simulink subsystem "HIL"  (R2024a)
settings: Solver=VariableStepAuto  StartTime=0.0  StopTime=10.0  RelTol=1e-3
values from neighbouring files (symbols this model uses):
  Hil = 100.0    [ModelDD.sldd]
  Sim : value not decoded    [ModelDD.sldd]
undefined symbols (not defined in the file or in its folder): D1, Delta, DiscIntNeverNeededParam
libraries: simulink x60, spsSeriesRLCBranchLib x18, spsControlledVoltageSourceLib x15, spsThreePhaseVIMeasurementLib x9, spsGroundLib x8, hdlsllib x6, spsMosfetLib x6, spsabctodq0Lib x5, spsDCVoltageSourceLib x3, spsPower3phInstantaneousLib x3, spsVoltageMeasurementLib x3, spspowerguiLib x3
(part 1 of 3)
settings Model: Creator=The Professionals  LastModifiedBy=The Professionals

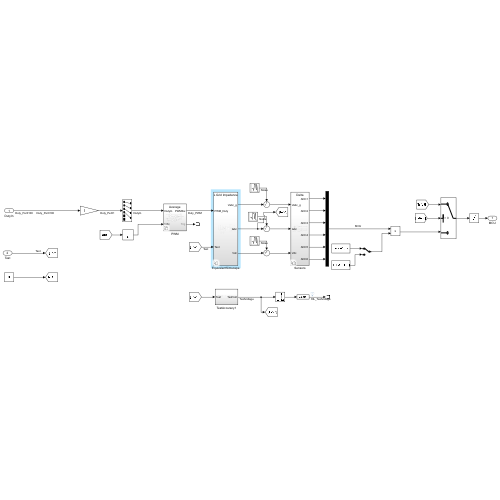
[thumbnail: Simulink's stored preview of the top-level diagram]
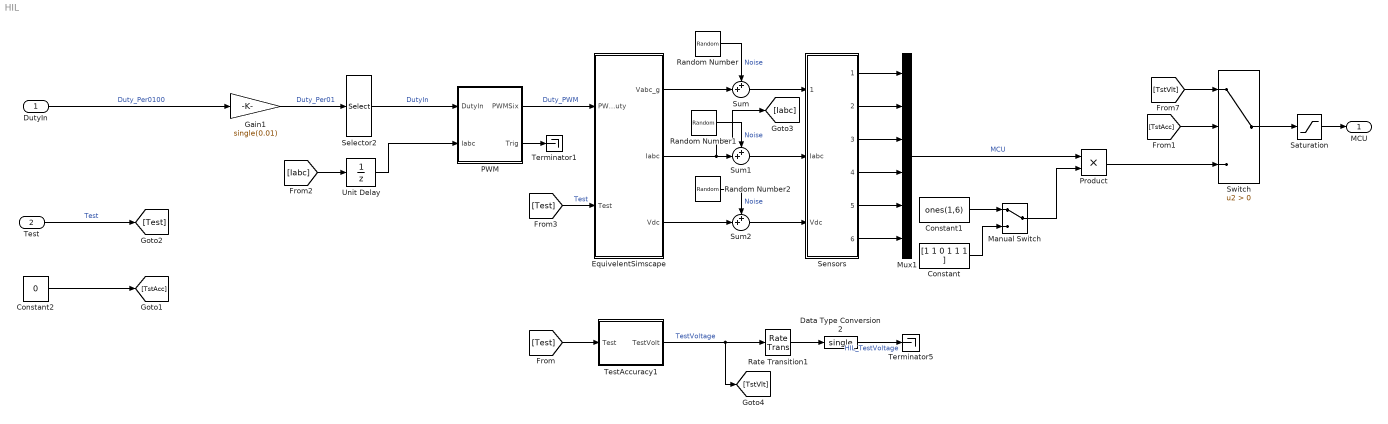
== system HIL ==
  DutyIn : Inport
  Test : Inport  Port=2
  Constant : Constant  Value=[1 1 0 1 1 1 ]
  Constant1 : Constant  Value=ones(1,6)
  Constant2 : Constant  Value=0  OutDataTypeStr=boolean
  Data Type Conversion2 : DataTypeConversion  OutDataTypeStr=single  SaturateOnIntegerOverflow=off  RndMeth=Floor
  EquivelentSimscape : Subsystem  Variant=on  VariantControl=EquivelentSimscape
  Gain1 : Gain  Gain=single(0.01)  ParamDataTypeStr=Inherit: Same as input
  Manual Switch : ManualSwitch
  Mux1 : Mux  Inputs=6
  PWM : Subsystem  Variant=on  VariantControl=PWM
  Product : Product
  Random Number : RandomNumber  Variance=Hil.ADC_VgnoiseStd.^2  SampleTime=Sim.ContSampleTime
  Random Number1 : RandomNumber  Variance=Hil.ADC_InoiseStd.^2  SampleTime=Sim.ContSampleTime
  Random Number2 : RandomNumber  Variance=Hil.ADC_VdcnoiseStd .^2  SampleTime=Sim.ContSampleTime
  Rate Transition1 : RateTransition  OutPortSampleTime=Hil.MeasSlowSmplTime
  Saturation : Saturate  UpperLimit=3  LowerLimit=0
  Selector2 : Selector  InputPortWidth=6  IndexOptions=Index vector (dialog)  Indices=[1 2 3 4]  OutputSizes=1
  Sensors : Subsystem  Variant=on  VariantControl=Scale
  Sum : Sum  Inputs=++|
  Sum1 : Sum  Inputs=++|
  Sum2 : Sum  Inputs=++|
  Switch : Switch  Criteria=u2 > Threshold  SaturateOnIntegerOverflow=off  InputSameDT=off
  Terminator1 : Terminator
  Terminator5 : Terminator
  TestAccuracy1 : Subsystem
  Unit Delay : UnitDelay  SampleTime=-1  HasFrameUpgradeWarning=on
  MCU : Outport  VectorParamsAs1DForOutWhenUnconnected=off
  wires:
  Gain1/1 -> Selector2/1  "Duty_Per01"
  DutyIn/1 -> Gain1/1  "Duty_Per0100"
  Test/1 -> [Test]  "Test"
  Random Number2/1 -> Sum2/1  "Noise"
  Manual Switch/1 -> Product/2
  Constant1/1 -> Manual Switch/1
  Sensors/4(ADC4) -> Mux1/4
  Random Number1/1 -> Sum1/1  "Noise"
  Random Number/1 -> Sum/1  "Noise"
  Sensors/1(ADC1) -> Mux1/1
  Constant/1 -> Manual Switch/2
  Sum2/1 -> Sensors/3(Vdc)
  Sensors/6(ADC6) -> Mux1/6
  Sum1/1 -> Sensors/2(Iabc)
  Mux1/1 -> Product/1  "MCU"
  Sensors/2(ADC2) -> Mux1/2
  Sum/1 -> Sensors/1(Vabc_g)
  Sensors/3(ADC3) -> Mux1/3
  Sensors/5(ADC5) -> Mux1/5
  [Test] -> EquivelentSimscape/2(Test)  "Test"
  EquivelentSimscape/1(Vabc_g) -> Sum/2
  EquivelentSimscape/2(Iabc) -> [Iabc], Sum1/2
  EquivelentSimscape/3(Vdc) -> Sum2/2
  Selector2/1 -> PWM/1(DutyIn)  "DutyIn"
  [Iabc] -> Unit Delay/1
  PWM/1(PWMSix) -> EquivelentSimscape/1(PWM_Duty)  "Duty_PWM"
  PWM/2(Trig) -> Terminator1/1
  Data Type Conversion2/1 -> Terminator5/1  "HIL_TestVoltage"
  TestAccuracy1/1(TestVolt) -> [TstVlt], Rate Transition1/1  "TestVoltage"
  [Test] -> TestAccuracy1/1(Test)
  Constant2/1 -> [TstAcc]
  Rate Transition1/1 -> Data Type Conversion2/1
  Switch/1 -> Saturation/1
  Saturation/1 -> MCU/1
  [TstVlt] -> Switch/1
  Product/1 -> Switch/3
  [TstAcc] -> Switch/2
  Unit Delay/1 -> PWM/2(Iabc)

== system HIL/EquivelentSimscape ==
  PWM_Duty : Inport
  Test : Inport  Port=2
  Continous : Subsystem  VariantControl="Sim.HilModel == \"Continous\""
  LGridImpedance : Subsystem  VariantControl="Sim.HilModel == \"LGridImp\""
  Taraz : Subsystem  VariantControl="Sim.HilModel == \"Taraz\""
  TarazAvg : Subsystem  VariantControl="Sim.HilModel == \"TarazAvg\""
  Vabc_g : Outport
  Iabc : Outport  Port=2
  Vdc : Outport  Port=3

== system HIL/PWM ==
  DutyIn : Inport
  Iabc : Inport  Port=2
  Average : Subsystem  VariantControl="Sim.PwmModel == \"Average\""
  PWM : Subsystem  VariantControl="Sim.PwmModel == \"PWM\""
  PWMSix : Outport
  Trig : Outport  Port=2

== system HIL/Sensors ==
  Vabc_g : Inport
  Iabc : Inport  Port=2
  Vdc : Inport  Port=3
  Delta : Subsystem  VariantControl="Sim.ADC_UabcSensor  ==  \"Three Currents\""
  Star : Subsystem  VariantControl="Sim.ADC_UabcSensor  == \"Three Volts\""
  ADC1 : Outport
  ADC2 : Outport  Port=2
  ADC3 : Outport  Port=3
  ADC4 : Outport  Port=4
  ADC5 : Outport  Port=5
  ADC6 : Outport  Port=6

== system HIL/TestAccuracy1 ==
  Test : Inport
  Compare To Constant : simulink/Logic and Bit Operations/Compare To Constant  relop=<  const=3.0  OutDataTypeStr=boolean
  Gain : Gain  Gain=3/50
  Gain5 : Gain  Gain=Sim.ContSampleTime  ParamDataTypeStr=double  OutDataTypeStr=double
  HDL Counter : hdlsllib/Sources/HDL Counter  CountType=Free running  CountInit=0  CountStep=1  CountMax=25  CountFromType=Initial value  CountFrom=0  CountResetPort=on  CountLoadPort=off  CountEnbPort=on  CountDirPort=off  CountHitOutputPort=off  CountDataType=Unsigned  CountWordLen=32  CountFracLen=0  CountSampTime=1
  NOT : Logic  Operator=NOT  AllPortsSameDT=off  OutDataTypeStr=boolean
  OR : Logic  AllPortsSameDT=off  OutDataTypeStr=boolean
  Round : Rounding  Operator=round
  Saturation : Saturate  UpperLimit=3  LowerLimit=0
  Unit Delay : UnitDelay  SampleTime=-1  HasFrameUpgradeWarning=on
  TestVolt : Outport
  wires:
  HDL Counter/1 -> Gain5/1
  Test/1 -> OR/1, NOT/1
  Gain/1 -> Saturation/1
  NOT/1 -> HDL Counter/1
  Round/1 -> Gain/1
  Saturation/1 -> Compare To Constant/1, TestVolt/1
  Compare To Constant/1 -> Unit Delay/1
  Unit Delay/1 -> OR/2
  Gain5/1 -> Round/1
  OR/1 -> HDL Counter/2

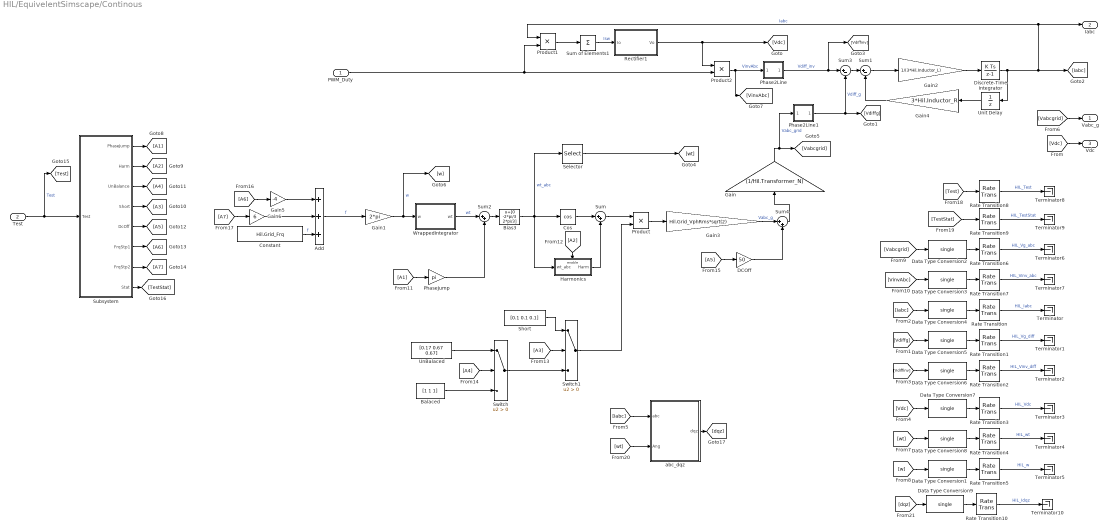
== system HIL/EquivelentSimscape/Continous ==
  PWM_Duty : Inport
  Test : Inport  Port=2
  Add : Sum  Inputs=+++
  Balaced : Constant  Value=[1 1 1]
  Bias3 : Bias  Bias=[0 -2*pi/3 2*pi/3]  SaturateOnIntegerOverflow=off
  Constant : Constant  Value=Hil.Grid_Frq
  Cos : Trigonometry  Operator=cos
  DCOff : Gain  Gain=50
  Data Type Conversion{1..9} (9 alike) : DataTypeConversion  OutDataTypeStr=single  SaturateOnIntegerOverflow=off  RndMeth=Floor
  Discrete-Time Integrator : DiscreteIntegrator  gainval=single(1)  InitialCondition=single(0)  SampleTime=-1  ICPrevOutput=DiscIntNeverNeededParam  ICPrevScaledInput=DiscIntNeverNeededParam
  Gain : Gain  Gain=(1/Hil.Transformer_N)
  Gain1 : Gain  Gain=2*pi
  Gain2 : Gain  Gain=1/(3*Hil.Inductor_L)
  Gain3 : Gain  Gain=Hil.Grid_VphRms*sqrt(2)
  Gain4 : Gain  Gain=3*Hil.Inductor_R
  Gain5 : Gain  Gain=-4
  Gain6 : Gain  Gain=6
  Harmonics : Subsystem
  Phase2Line : Subsystem
  Phase2Line1 : Subsystem
  PhaseJump : Gain  Gain=pi
  Product : Product
  Product1 : Product
  Product2 : Product
  Rate Transition{,1..10} (11 alike) : RateTransition  OutPortSampleTime=1/10000
  Rectifier1 : Subsystem
  Selector : Selector  InputPortWidth=3  IndexOptions=Index vector (dialog)  Indices=[1]  OutputSizes=1
  Short : Constant  Value=[0.1 0.1 0.1]
  Subsystem : Subsystem
  Sum : Sum  Inputs=|++
  Sum of Elements1 : Sum  Inputs=+
  Sum1 : Sum  Inputs=|+-
  Sum2 : Sum  Inputs=|++
  Sum3 : Sum  Inputs=|+-
  Sum4 : Sum  Inputs=|++
  Switch : Switch  Criteria=u2 > Threshold  SaturateOnIntegerOverflow=off  InputSameDT=off
  Switch1 : Switch  Criteria=u2 > Threshold  SaturateOnIntegerOverflow=off  InputSameDT=off
  Terminator{,1..10} (11 alike) : Terminator
  UnBalaced : Constant  Value=[0.17 0.67 0.67]
  Unit Delay : UnitDelay  SampleTime=-1  HasFrameUpgradeWarning=on
  WrappedIntegrator : Subsystem
  abc_dqz : Subsystem  VariantControl=Var.Pll.SOGISel == 2
  Vabc_g : Outport
  Iabc : Outport  Port=2
  Vdc : Outport  Port=3
  wires:
  [dqz] -> Data Type Conversion9/1
  Data Type Conversion9/1 -> Rate Transition10/1
  Rate Transition10/1 -> Terminator10/1  "HIL_Idqz"
  abc_dqz/1(dqz) -> [dqz]
  [wt] -> abc_dqz/2(Ang)
  [Iabc] -> abc_dqz/1(abc)
  [TestStat] -> Rate Transition9/1
  Rate Transition9/1 -> Terminator9/1  "HIL_TestStat"
  Subsystem/8(Stat) -> [TestStat]
  [Test] -> Rate Transition8/1
  Rate Transition8/1 -> Terminator8/1  "HIL_Test"
  [A7] -> Gain6/1
  Subsystem/7(FrqStp2) -> [A7]
  [A6] -> Gain5/1
  Subsystem/6(FrqStp1) -> [A6]
  Gain5/1 -> Add/1
  Gain6/1 -> Add/2
  Constant/1 -> Add/3  "f"
  [A5] -> DCOff/1
  Subsystem/5(DcOff) -> [A5]
  DCOff/1 -> Sum4/2
  [A4] -> Switch/2
  Subsystem/3(UnBalance) -> [A4]
  [A3] -> Switch1/2
  Subsystem/4(Short) -> [A3]
  Short/1 -> Switch1/1
  Switch/1 -> Switch1/3
  UnBalaced/1 -> Switch/1
  Balaced/1 -> Switch/3
  [A2] -> Harmonics/Enable
  Subsystem/2(Harm) -> [A2]
  [A1] -> PhaseJump/1
  Subsystem/1(PhaseJump) -> [A1]
  Test/1 -> Subsystem/1(Test), [Test]  "Test"
  PhaseJump/1 -> Sum2/2
  [VinvAbc] -> Data Type Conversion3/1
  [Vabcgrid] -> Data Type Conversion2/1
  Rate Transition6/1 -> Terminator6/1  "HIL_Vg_abc"
  Rate Transition7/1 -> Terminator7/1  "HIL_Vinv_abc"
  Data Type Conversion2/1 -> Rate Transition6/1
  Data Type Conversion3/1 -> Rate Transition7/1
  Sum4/1 -> Gain/1
  Switch1/1 -> Product/2
  Sum/1 -> Product/1
  Sum2/1 -> Bias3/1
  Harmonics/1(Harm) -> Sum/2
  Product/1 -> Gain3/1
  Bias3/1 -> Harmonics/1(wt_abc), Selector/1, Cos/1  "wt_abc"
  Selector/1 -> [wt]
  [w] -> Data Type Conversion1/1
  Rate Transition5/1 -> Terminator5/1  "HIL_w"
  Data Type Conversion1/1 -> Rate Transition5/1
  Rate Transition4/1 -> Terminator4/1  "HIL_wt"
  Data Type Conversion8/1 -> Rate Transition4/1
  Data Type Conversion7/1 -> Rate Transition3/1
  Data Type Conversion6/1 -> Rate Transition2/1
  Data Type Conversion5/1 -> Rate Transition1/1
  Data Type Conversion4/1 -> Rate Transition/1
  [wt] -> Data Type Conversion8/1
  [Vabcgrid] -> Vabc_g/1
  [Vdc] -> Data Type Conversion7/1
  Rate Transition3/1 -> Terminator3/1  "HIL_Vdc"
  Rate Transition2/1 -> Terminator2/1  "HIL_Vinv_diff"
  Rate Transition1/1 -> Terminator1/1  "HIL_Vg_diff"
  [Vdiffinv] -> Data Type Conversion6/1
  [Iabc] -> Data Type Conversion4/1
  [Vdiffg] -> Data Type Conversion5/1
  Rate Transition/1 -> Terminator/1  "HIL_Iabc"
  Sum of Elements1/1 -> Rectifier1/1(Io)  "Isw"
  Product2/1 -> [VinvAbc], Phase2Line/1(In1)  "VinvAbc"
  PWM_Duty/1 -> Product1/2, Product2/2
  [Vdc] -> Vdc/1
  Gain/1 -> Phase2Line1/1(In1), [Vabcgrid]  "Vabc_grid"
  Product1/1 -> Sum of Elements1/1
  Rectifier1/1(Vo) -> Product2/1, [Vdc]
  Gain4/1 -> Sum1/2
  Unit Delay/1 -> Gain4/1
  Sum1/1 -> Gain2/1
  Phase2Line1/1(Out1) -> [Vdiffg], Sum3/2  "Vdiff_g"
  Cos/1 -> Sum/1
  WrappedIntegrator/1(wt) -> Sum2/1  "wt"
  Gain1/1 -> WrappedIntegrator/1(w), [w]  "w"
  Discrete-Time Integrator/1 -> Product1/1, Iabc/1, [Iabc], Unit Delay/1  "Iabc"
  Gain2/1 -> Discrete-Time Integrator/1
  Sum3/1 -> Sum1/1
  Gain3/1 -> Sum4/1  "Vabc_g"
  Add/1 -> Gain1/1  "f"
  Phase2Line/1(Out1) -> [Vdiffinv], Sum3/1  "Vdiff_inv"

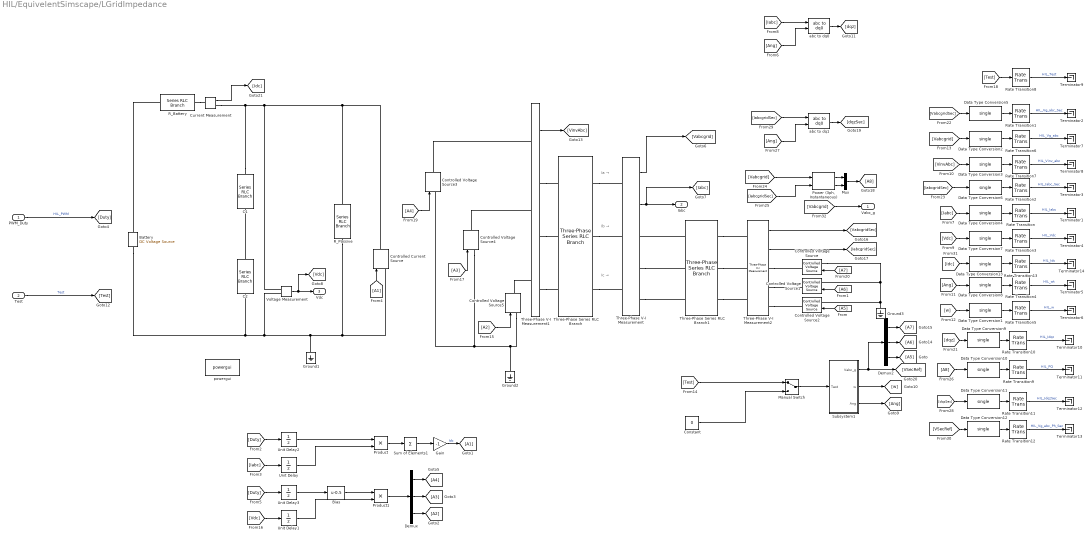
== system HIL/EquivelentSimscape/LGridImpedance ==
  note: Ia
      | →
  note: Ib
      | →
  note: Ic
      | →
  PWM_Duty : Inport
  Test : Inport  Port=2
  Battery : spsDCVoltageSourceLib/DC Voltage Source  Amplitude=Hil.HVDC_V  Measurements=None
  Bias : Bias  Bias=-0.5  SaturateOnIntegerOverflow=off
  C1 : spsSeriesRLCBranchLib/Series RLC Branch  LConnTagsString=__new0  RConnTagsString=__new0  BranchType=RLC  Resistance=Hil.HVDC_Cesr  Inductance=Hil.HVDC_Cesl  SetiL0=off  InitialCurrent=0  Capacitance=Hil.HVDC_C/2  Setx0=off  InitialVoltage=0  Measurements=None
  C2 : spsSeriesRLCBranchLib/Series RLC Branch  LConnTagsString=__new0  RConnTagsString=__new0  BranchType=RLC  Resistance=Hil.HVDC_Cesr  Inductance=Hil.HVDC_Cesl  SetiL0=off  InitialCurrent=0  Capacitance=Hil.HVDC_C/2  Setx0=off  InitialVoltage=0  Measurements=None
  Constant : Constant  Value=0  OutDataTypeStr=boolean
  Controlled Current Source : spsControlledCurrentSourceLib/Controlled Current Source  Initialize=on  Source_Type=AC  Amplitude=0  Phase=0  Frequency=0  Measurements=None
  Controlled Voltage Source{,1..5} (6 alike) : spsControlledVoltageSourceLib/Controlled Voltage Source  Initialize=on  Source_Type=AC  Amplitude=0  Phase=0  Frequency=0  Measurements=None
  Current Measurement : spsCurrentMeasurementLib/Current Measurement  PhasorSimulation=off  OutputType=Complex  PSBequivalent=0
  Data Type Conversion{1..13} (13 alike) : DataTypeConversion  OutDataTypeStr=single  SaturateOnIntegerOverflow=off  RndMeth=Floor
  Demux : Demux  Outputs=3
  Demux2 : Demux  Outputs=3
  Gain : Gain  Gain=-1
  Ground1 : spsGroundLib/Ground  LConnTagsString=a
  Ground2 : spsGroundLib/Ground  LConnTagsString=a
  Ground3 : spsGroundLib/Ground  LConnTagsString=a
  Manual Switch : ManualSwitch
  Mux : Mux  Inputs=2
  "Power (3ph, Instantaneous)" : spsPower3phInstantaneousLib/Power (3ph, Instantaneous)
  Product : Product
  Product1 : Product
  R_Battery : spsSeriesRLCBranchLib/Series RLC Branch  LConnTagsString=__new0  RConnTagsString=__new0  BranchType=R  Resistance=Hil.HVDC_Vesr  Inductance=Hil.HVDC_Vesl  SetiL0=off  InitialCurrent=0  Capacitance=1e-6  Setx0=off  InitialVoltage=0  Measurements=None
  R_Passive : spsSeriesRLCBranchLib/Series RLC Branch  LConnTagsString=__new0  RConnTagsString=__new0  BranchType=R  Resistance=Hil.HVDC_Rpasiv  Inductance=1e-3  SetiL0=off  InitialCurrent=0  Capacitance=1e-6  Setx0=off  InitialVoltage=0  Measurements=None
  Rate Transition{,1..2,4,6..7,12} (7 alike) : RateTransition  OutPortSampleTime=Hil.MeasFastSmplTime
  Rate Transition{3,5,8..11,13} (7 alike) : RateTransition  OutPortSampleTime=Hil.MeasSlowSmplTime
  Subsystem1 : Subsystem
  Sum of Elements1 : Sum  Inputs=+
  Terminator{1..14} (14 alike) : Terminator
  Three-Phase Series RLC Branch : spsThreePhaseSeriesRLCBranchLib/Three-Phase Series RLC Branch  LConnTagsString=A|B|C  RConnTagsString=A|B|C  BranchType=RL  Resistance=Hil.Inductor_R  Inductance=Hil.Inductor_L  Capacitance=1e-6  Measurements=None
  Three-Phase Series RLC Branch1 : spsThreePhaseSeriesRLCBranchLib/Three-Phase Series RLC Branch  LConnTagsString=A|B|C  RConnTagsString=A|B|C  BranchType=RL  Resistance=Hil.Inductor_Rg  Inductance=Hil.Inductor_Lg  Capacitance=1e-6  Measurements=None
  Three-Phase V-I Measurement : spsThreePhaseVIMeasurementLib/Three-Phase V-I Measurement  VoltageMeasurement=phase-to-ground  SetLabelV=off  LabelV=Vabc  Vpu=off  VpuLL=off  CurrentMeasurement=yes  SetLabelI=off  LabelI=Iabc  Ipu=off  Pbase=100e6  Vbase=500e3  OutputType=Complex  PhasorSimulation=off  PSBequivalent=0
  Three-Phase V-I Measurement1 : spsThreePhaseVIMeasurementLib/Three-Phase V-I Measurement  VoltageMeasurement=phase-to-ground  SetLabelV=off  LabelV=Vabc  Vpu=off  VpuLL=off  CurrentMeasurement=no  SetLabelI=off  LabelI=Iabc  Ipu=off  Pbase=100e6  Vbase=500e3  OutputType=Complex  PhasorSimulation=off  PSBequivalent=0
  Three-Phase V-I Measurement2 : spsThreePhaseVIMeasurementLib/Three-Phase V-I Measurement  VoltageMeasurement=phase-to-ground  SetLabelV=off  LabelV=Vabc  Vpu=off  VpuLL=off  CurrentMeasurement=yes  SetLabelI=off  LabelI=Iabc  Ipu=off  Pbase=100e6  Vbase=500e3  OutputType=Complex  PhasorSimulation=off  PSBequivalent=0
  Unit Delay{,1..3} (4 alike) : UnitDelay  SampleTime=-1  HasFrameUpgradeWarning=on
  Voltage Measurement : spsVoltageMeasurementLib/Voltage Measurement  PhasorSimulation=off  OutputType=Complex  PSBequivalent=0
  abc to dq0 : spsabctodq0Lib/abc to dq0  Alignment=Aligned with phase A axis
  abc to dq1 : spsabctodq0Lib/abc to dq0  Alignment=Aligned with phase A axis
  powergui : spspowerguiLib/powergui  Priority=1  SimulationMode=Discrete  SampleTime=Sim.ContSampleTime  frequency=60  Iterations=50  frequencyindice=0  Pbase=100e6  ErrMax=1e-4  UnitsV=kV  UnitsW=MW  buscounter=0  FunctionMessages=off  echomessages=off  EnableUseOfTLC=off  CurrentSourceSwitches=off  DisableSnubberDevices=off  DisableRonSwitches=off  DisableVfSwitches=off  DisplayEquations=off  AutomaticDiscreteSolvers=off  SolverType=Tustin/Backward Euler (TBE)  Interpol=off  ExternalGateDelay=off  methode=off  Ts=100  x0status=blocks  SPID=on  SwTol=0  HookPort=off  NonlinearTolerance=1e-4  nMaxIteration=100  ContinueOnMaxIteration=off  RestoreLinks=warning  ResistiveCurrentMeasurement=off  Frange=[0:2:500]  Ylog=off  Xlog=on  ShowGrid=off  save=off  variable=ZData  structure=0  ZoomFFT=off  StartTime=0.0  cycles=1  DisplayStyle=1  fundamental=60  FreqAxis=off  MaxFrequency=1000  frequencyindicesteady=1  RmsSteady=1  display=off
  Vabc_g : Outport
  Iabc : Outport  Port=2
  Vdc : Outport  Port=3
  wires:
  [Idc] -> Data Type Conversion13/1
  Rate Transition13/1 -> Terminator14/1  "HIL_Idc"
  Data Type Conversion13/1 -> Rate Transition13/1
  Current Measurement/1 -> [Idc]
  [VSecRef] -> Data Type Conversion12/1
  Data Type Conversion12/1 -> Rate Transition12/1
  Rate Transition12/1 -> Terminator13/1  "HIL_Vg_abc_Ph_Sec"
  [dqzSec] -> Data Type Conversion11/1
  Rate Transition11/1 -> Terminator12/1  "HIL_IdqzSec"
  Data Type Conversion11/1 -> Rate Transition11/1
  [IabcgridSec] -> abc to dq1/1
  abc to dq1/1 -> [dqzSec]
  [Ang] -> abc to dq1/2
  [A8] -> Data Type Conversion10/1
  Mux/1 -> [A8]
  Rate Transition9/1 -> Terminator11/1  "HIL_PQ"
  Data Type Conversion10/1 -> Rate Transition9/1
  "Power (3ph, Instantaneous)"/2 -> Mux/2
  "Power (3ph, Instantaneous)"/1 -> Mux/1
  [IabcgridSec] -> "Power (3ph, Instantaneous)"/2
  [Vabcgrid] -> "Power (3ph, Instantaneous)"/1
  [IabcgridSec] -> Data Type Conversion6/1
  Rate Transition2/1 -> Terminator3/1  "HIL_Iabc_Sec"
  Data Type Conversion6/1 -> Rate Transition2/1
  [VabcgridSec] -> Data Type Conversion5/1
  Rate Transition1/1 -> Terminator2/1  "HIL_Vg_abc_Sec"
  Data Type Conversion5/1 -> Rate Transition1/1
  Three-Phase V-I Measurement2/2 -> [IabcgridSec]
  Three-Phase V-I Measurement2/1 -> [VabcgridSec]
  [A7] -> Controlled Voltage Source/1
  Demux2/1 -> [A7]
  [A6] -> Controlled Voltage Source1/1
  Demux2/2 -> [A6]
  [A5] -> Controlled Voltage Source2/1
  Demux2/3 -> [A5]
  [Test] -> Manual Switch/1
  Constant/1 -> Manual Switch/2
  Unit Delay3/1 -> Bias/1
  Unit Delay2/1 -> Product/1
  Subsystem1/3(Ang) -> [Ang]
  Subsystem1/2(w) -> [w]
  Manual Switch/1 -> Subsystem1/1(Test)
  Three-Phase V-I Measurement1/1 -> [VinvAbc]
  Test/1 -> [Test]  "Test"
  Three-Phase V-I Measurement/1 -> [Vabcgrid]
  Three-Phase V-I Measurement/2 -> [Iabc], Iabc/1
  Voltage Measurement/1 -> [Vdc], Vdc/1
  PWM_Duty/1 -> [Duty]  "HIL_PWM"
  [Vdc] -> Data Type Conversion7/1
  [dqz] -> Data Type Conversion9/1
  Data Type Conversion9/1 -> Rate Transition10/1
  Rate Transition8/1 -> Terminator9/1  "HIL_Test"
  Data Type Conversion2/1 -> Rate Transition6/1
  [Test] -> Rate Transition8/1
  [VinvAbc] -> Data Type Conversion3/1
  Data Type Conversion4/1 -> Rate Transition/1
  Data Type Conversion8/1 -> Rate Transition4/1
  Data Type Conversion3/1 -> Rate Transition7/1
  Rate Transition6/1 -> Terminator7/1  "HIL_Vg_abc"
  [Vabcgrid] -> Data Type Conversion2/1
  Rate Transition7/1 -> Terminator8/1  "HIL_Vinv_abc"
  Data Type Conversion1/1 -> Rate Transition5/1
  [Ang] -> Data Type Conversion8/1
  Rate Transition4/1 -> Terminator5/1  "HIL_wt"
  Rate Transition10/1 -> Terminator10/1  "HIL_Idqz"
  Data Type Conversion7/1 -> Rate Transition3/1
  Rate Transition3/1 -> Terminator4/1  "HIL_Vdc"
  [Iabc] -> Data Type Conversion4/1
  Rate Transition/1 -> Terminator1/1  "HIL_Iabc"
  [w] -> Data Type Conversion1/1
  Rate Transition5/1 -> Terminator6/1  "HIL_w"
  [Ang] -> abc to dq0/2
  abc to dq0/1 -> [dqz]
  [Iabc] -> abc to dq0/1
  Subsystem1/1(Vabc_g) -> Demux2/1, [VSecRef]
  [Duty] -> Unit Delay2/1
  [Iabc] -> Unit Delay/1
  Product/1 -> Sum of Elements1/1
  Unit Delay/1 -> Product/2
  Sum of Elements1/1 -> Gain/1
  Gain/1 -> [A1]  "Idc"
  [A1] -> Controlled Current Source/1
  Unit Delay1/1 -> Product1/2
  Product1/1 -> Demux/1
  [Vdc] -> Unit Delay1/1
  [Duty] -> Unit Delay3/1
  Demux/3 -> [A2]
  [A2] -> Controlled Voltage Source5/1
  Demux/2 -> [A3]
  [A3] -> Controlled Voltage Source4/1
  Demux/1 -> [A4]
  [A4] -> Controlled Voltage Source3/1
  Bias/1 -> Product1/1
  [Vabcgrid] -> Vabc_g/1
  connections:
  Three-Phase V-I Measurement1/RConn1 -- Three-Phase Series RLC Branch/LConn1
  Three-Phase V-I Measurement1/RConn2 -- Three-Phase Series RLC Branch/LConn2
  Three-Phase V-I Measurement1/RConn3 -- Three-Phase Series RLC Branch/LConn3
  R_Battery/RConn1 -- Current Measurement/LConn1
  C1/LConn1 -- Current Measurement/RConn1 -- Voltage Measurement/LConn1 -- Controlled Current Source/RConn1 -- R_Passive/LConn1
  Three-Phase V-I Measurement2/RConn1 -- Controlled Voltage Source/RConn1
  Three-Phase V-I Measurement2/RConn2 -- Controlled Voltage Source1/RConn1
  Three-Phase V-I Measurement2/RConn3 -- Controlled Voltage Source2/RConn1
  Three-Phase Series RLC Branch1/RConn3 -- Three-Phase V-I Measurement2/LConn3
  Three-Phase Series RLC Branch1/RConn2 -- Three-Phase V-I Measurement2/LConn2
  Three-Phase Series RLC Branch1/RConn1 -- Three-Phase V-I Measurement2/LConn1
  Battery/RConn1 -- R_Battery/LConn1
  C2/LConn1 -- C1/RConn1
  R_Passive/RConn1 -- Voltage Measurement/LConn2 -- Battery/LConn1 -- C2/RConn1 -- Ground1/LConn1 -- Controlled Current Source/LConn1
  Three-Phase Series RLC Branch/RConn2 -- Three-Phase V-I Measurement/LConn2
  Three-Phase Series RLC Branch/RConn3 -- Three-Phase V-I Measurement/LConn3
  Three-Phase Series RLC Branch/RConn1 -- Three-Phase V-I Measurement/LConn1
  Three-Phase V-I Measurement/RConn3 -- Three-Phase Series RLC Branch1/LConn3
  Three-Phase V-I Measurement/RConn2 -- Three-Phase Series RLC Branch1/LConn2
  Three-Phase Series RLC Branch1/LConn1 -- Three-Phase V-I Measurement/RConn1
  Controlled Voltage Source2/LConn1 -- Ground3/LConn1 -- Controlled Voltage Source1/LConn1 -- Controlled Voltage Source/LConn1
  Controlled Voltage Source5/RConn1 -- Three-Phase V-I Measurement1/LConn3
  Controlled Voltage Source4/RConn1 -- Three-Phase V-I Measurement1/LConn2
  Three-Phase V-I Measurement1/LConn1 -- Controlled Voltage Source3/RConn1
  Controlled Voltage Source4/LConn1 -- Controlled Voltage Source5/LConn1 -- Ground2/LConn1 -- Controlled Voltage Source3/LConn1

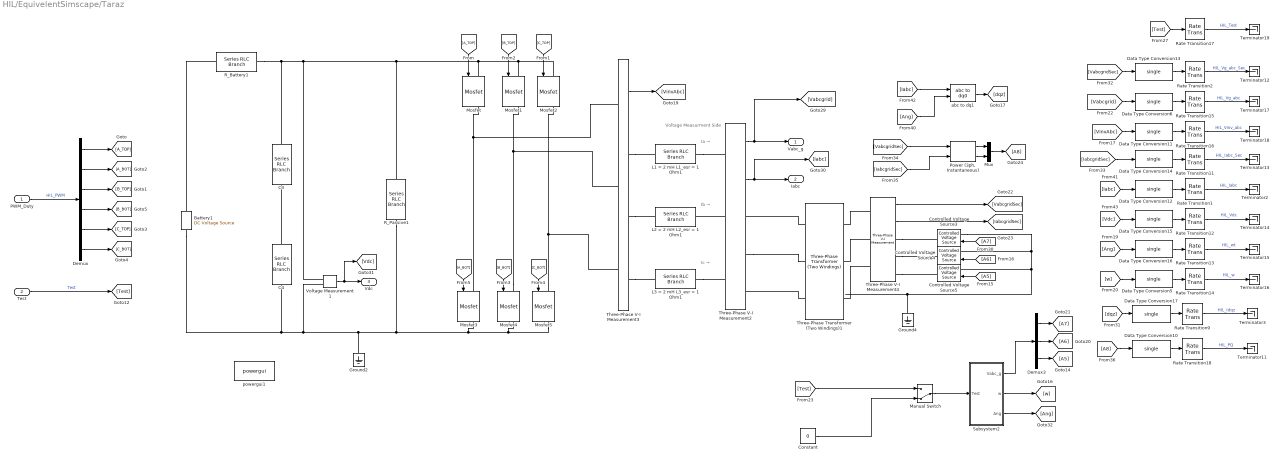
== system HIL/EquivelentSimscape/Taraz ==
  note: Voltage
      | Measurment
      | Side
  note: Ib
      | →
  note: Ic
      | →
  note: Ia
      | →
  PWM_Duty : Inport
  Test : Inport  Port=2
  Battery1 : spsDCVoltageSourceLib/DC Voltage Source  Amplitude=Hil.HVDC_V  Measurements=None
  C3 : spsSeriesRLCBranchLib/Series RLC Branch  LConnTagsString=__new0  RConnTagsString=__new0  BranchType=RLC  Resistance=Hil.HVDC_Cesr  Inductance=Hil.HVDC_Cesl  SetiL0=off  InitialCurrent=0  Capacitance=Hil.HVDC_C/2  Setx0=off  InitialVoltage=0  Measurements=None
  C4 : spsSeriesRLCBranchLib/Series RLC Branch  LConnTagsString=__new0  RConnTagsString=__new0  BranchType=RLC  Resistance=Hil.HVDC_Cesr  Inductance=Hil.HVDC_Cesl  SetiL0=off  InitialCurrent=0  Capacitance=Hil.HVDC_C/2  Setx0=off  InitialVoltage=0  Measurements=None
  Constant : Constant  Value=0  OutDataTypeStr=boolean
  Controlled Voltage Source3 : spsControlledVoltageSourceLib/Controlled Voltage Source  Initialize=on  Source_Type=AC  Amplitude=0  Phase=0  Frequency=0  Measurements=None
  Controlled Voltage Source4 : spsControlledVoltageSourceLib/Controlled Voltage Source  Initialize=on  Source_Type=AC  Amplitude=0  Phase=0  Frequency=0  Measurements=None
  Controlled Voltage Source5 : spsControlledVoltageSourceLib/Controlled Voltage Source  Initialize=on  Source_Type=AC  Amplitude=0  Phase=0  Frequency=0  Measurements=None
  Data Type Conversion{5..6,10..17} (10 alike) : DataTypeConversion  OutDataTypeStr=single  SaturateOnIntegerOverflow=off  RndMeth=Floor
  Demux : Demux  Outputs=6
  Demux3 : Demux  Outputs=3
  Ground2 : spsGroundLib/Ground  LConnTagsString=a
  Ground4 : spsGroundLib/Ground  LConnTagsString=a
  L1 = 2 mH L1_esr = 1 Ohm1 : spsSeriesRLCBranchLib/Series RLC Branch  LConnTagsString=__new0  RConnTagsString=__new0  BranchType=RL  Resistance=Hil.Inductor_R  Inductance=Hil.Inductor_L  SetiL0=off  InitialCurrent=0  Capacitance=1e-6  Setx0=off  InitialVoltage=0  Measurements=None
  L2 = 2 mH L2_esr = 1 Ohm1 : spsSeriesRLCBranchLib/Series RLC Branch  LConnTagsString=__new0  RConnTagsString=__new0  BranchType=RL  Resistance=Hil.Inductor_R  Inductance=Hil.Inductor_L  SetiL0=off  InitialCurrent=0  Capacitance=1e-6  Setx0=off  InitialVoltage=0  Measurements=None
  L3 = 2 mH L3_esr = 1 Ohm1 : spsSeriesRLCBranchLib/Series RLC Branch  LConnTagsString=__new0  RConnTagsString=__new0  BranchType=RL  Resistance=Hil.Inductor_R  Inductance=Hil.Inductor_L  SetiL0=off  InitialCurrent=0  Capacitance=1e-6  Setx0=off  InitialVoltage=0  Measurements=None
  Manual Switch : ManualSwitch  CurrentSetting=0
  Mosfet{,1..5} (6 alike) : spsMosfetLib/Mosfet  Ron=Hil.Sic_Ron  Lon=0  Rd=Hil.Sic_Rdiode  Vfd=Hil.Sic_Vdiode  IC=0  Rs=1e6  Cs=inf  Measurements=off
  Mux : Mux  Inputs=2
  "Power (3ph, Instantaneous)" : spsPower3phInstantaneousLib/Power (3ph, Instantaneous)
  R_Battery1 : spsSeriesRLCBranchLib/Series RLC Branch  LConnTagsString=__new0  RConnTagsString=__new0  BranchType=R  Resistance=Hil.HVDC_Vesr  Inductance=Hil.HVDC_Vesl  SetiL0=off  InitialCurrent=0  Capacitance=1e-6  Setx0=off  InitialVoltage=0  Measurements=None
  R_Passive1 : spsSeriesRLCBranchLib/Series RLC Branch  LConnTagsString=__new0  RConnTagsString=__new0  BranchType=R  Resistance=Hil.HVDC_Rpasiv  Inductance=1e-3  SetiL0=off  InitialCurrent=0  Capacitance=1e-6  Setx0=off  InitialVoltage=0  Measurements=None
  Rate Transition{1..2,11,13,15..16} (6 alike) : RateTransition  OutPortSampleTime=Hil.MeasFastSmplTime
  Rate Transition{9,12,14,17..18} (5 alike) : RateTransition  OutPortSampleTime=Hil.MeasSlowSmplTime
  Subsystem2 : Subsystem
  Terminator{2..3,11..19} (11 alike) : Terminator
  Three-Phase Transformer (Two Windings)1 : spsThreePhaseTransformerTwoWindingsLib/Three-Phase Transformer (Two Windings)  Winding1Connection=Delta (D1)  Winding2Connection=Yn  CoreType=Three single-phase transformers  SetSaturation=off  Hysteresis=off  DataFile='hysteresis'  SetInitialFlux=off  Measurements=None  UNITS=SI  NominalPower=[ 100e3 , 50 ]  Winding1=[100 Hil.Transformer_R1 Hil.Transformer_L1]  Winding2=[(Hil.Transformer_N )*100 Hil.Transformer_R2*(Hil.Transformer_N )^2 Hil.Transformer_R2*(Hil.Transformer_N )^2]  Rm=Hil.Transformer_Rc  Lm=Hil.Transformer_Lm  L0=0.5  Saturation=[0 0;1.1327 0.53955;471.96 0.68343]  InitialFluxes=[0.3597 -0.3597 0.31474]  BreakLoop=off  DiscreteSolver=Trapezoidal iterative  DataType=on  TransfoNumber=1
  Three-Phase V-I Measurement2 : spsThreePhaseVIMeasurementLib/Three-Phase V-I Measurement  VoltageMeasurement=phase-to-phase  SetLabelV=off  LabelV=Vabc  Vpu=off  VpuLL=off  CurrentMeasurement=yes  SetLabelI=off  LabelI=Iabc  Ipu=off  Pbase=100e6  Vbase=500e3  OutputType=Complex  PhasorSimulation=off  PSBequivalent=0
  Three-Phase V-I Measurement3 : spsThreePhaseVIMeasurementLib/Three-Phase V-I Measurement  VoltageMeasurement=phase-to-ground  SetLabelV=off  LabelV=Vabc  Vpu=off  VpuLL=off  CurrentMeasurement=no  SetLabelI=off  LabelI=Iabc  Ipu=off  Pbase=100e6  Vbase=500e3  OutputType=Complex  PhasorSimulation=off  PSBequivalent=0
  Three-Phase V-I Measurement4 : spsThreePhaseVIMeasurementLib/Three-Phase V-I Measurement  VoltageMeasurement=phase-to-phase  SetLabelV=off  LabelV=Vabc  Vpu=off  VpuLL=off  CurrentMeasurement=yes  SetLabelI=off  LabelI=Iabc  Ipu=off  Pbase=100e6  Vbase=500e3  OutputType=Complex  PhasorSimulation=off  PSBequivalent=0
  Voltage Measurement1 : spsVoltageMeasurementLib/Voltage Measurement  PhasorSimulation=off  OutputType=Complex  PSBequivalent=0
  abc to dq1 : spsabctodq0Lib/abc to dq0  Alignment=Aligned with phase A axis
  powergui1 : spspowerguiLib/powergui  Priority=1  SimulationMode=Discrete  SampleTime=Sim.ContSampleTime  frequency=60  Iterations=50  frequencyindice=0  Pbase=100e6  ErrMax=1e-4  UnitsV=kV  UnitsW=MW  buscounter=0  FunctionMessages=off  echomessages=off  EnableUseOfTLC=off  CurrentSourceSwitches=off  DisableSnubberDevices=off  DisableRonSwitches=off  DisableVfSwitches=off  DisplayEquations=off  AutomaticDiscreteSolvers=off  SolverType=Tustin/Backward Euler (TBE)  Interpol=off  ExternalGateDelay=off  methode=off  Ts=100  x0status=blocks  SPID=on  SwTol=0  HookPort=off  NonlinearTolerance=1e-4  nMaxIteration=100  ContinueOnMaxIteration=off  RestoreLinks=warning  ResistiveCurrentMeasurement=off  Frange=[0:2:500]  Ylog=off  Xlog=on  ShowGrid=off  save=off  variable=ZData  structure=0  ZoomFFT=off  StartTime=0.0  cycles=1  DisplayStyle=1  fundamental=60  FreqAxis=off  MaxFrequency=1000  frequencyindicesteady=1  RmsSteady=1  display=off
  Vabc_g : Outport
  Iabc : Outport  Port=2
  Vdc : Outport  Port=3
  wires:
  [w] -> Data Type Conversion5/1
  [A6] -> Controlled Voltage Source4/1
  [VabcgridSec] -> "Power (3ph, Instantaneous)"/1
  [A5] -> Controlled Voltage Source5/1
  Data Type Conversion12/1 -> Rate Transition1/1
  Demux3/2 -> [A6]
  Rate Transition1/1 -> Terminator2/1  "HIL_Iabc"
  Rate Transition16/1 -> Terminator18/1  "HIL_Vinv_abc"
  abc to dq1/1 -> [dqz]
  Rate Transition15/1 -> Terminator17/1  "HIL_Vg_abc"
  Data Type Conversion11/1 -> Rate Transition16/1
  [Iabc] -> abc to dq1/1
  Rate Transition9/1 -> Terminator3/1  "HIL_Idqz"
  [Iabc] -> Data Type Conversion12/1
  Rate Transition13/1 -> Terminator15/1  "HIL_wt"
  Subsystem2/1(Vabc_g) -> Demux3/1
  [Vabcgrid] -> Data Type Conversion6/1
  Rate Transition14/1 -> Terminator16/1  "HIL_w"
  [Ang] -> Data Type Conversion16/1
  Data Type Conversion5/1 -> Rate Transition14/1
  [VinvAbc] -> Data Type Conversion11/1
  Data Type Conversion6/1 -> Rate Transition15/1
  [dqz] -> Data Type Conversion17/1
  Three-Phase V-I Measurement2/2 -> [Iabc], Iabc/1
  Data Type Conversion15/1 -> Rate Transition12/1
  [Ang] -> abc to dq1/2
  Data Type Conversion17/1 -> Rate Transition9/1
  Voltage Measurement1/1 -> [Vdc], Vdc/1
  Three-Phase V-I Measurement3/1 -> [VinvAbc]
  Data Type Conversion16/1 -> Rate Transition13/1
  Rate Transition12/1 -> Terminator14/1  "HIL_Vdc"
  [Vdc] -> Data Type Conversion15/1
  Three-Phase V-I Measurement2/1 -> [Vabcgrid], Vabc_g/1
  Subsystem2/2(w) -> [w]
  Rate Transition2/1 -> Terminator12/1  "HIL_Vg_abc_Sec"
  Subsystem2/3(Ang) -> [Ang]
  Rate Transition17/1 -> Terminator19/1  "HIL_Test"
  [Test] -> Rate Transition17/1
  [A8] -> Data Type Conversion10/1
  Data Type Conversion10/1 -> Rate Transition18/1
  Rate Transition18/1 -> Terminator11/1  "HIL_PQ"
  Three-Phase V-I Measurement4/1 -> [VabcgridSec]
  Data Type Conversion13/1 -> Rate Transition2/1
  [IabcgridSec] -> Data Type Conversion14/1
  Manual Switch/1 -> Subsystem2/1(Test)
  Constant/1 -> Manual Switch/2
  [Test] -> Manual Switch/1
  [IabcgridSec] -> "Power (3ph, Instantaneous)"/2
  Mux/1 -> [A8]
  Data Type Conversion14/1 -> Rate Transition11/1
  Rate Transition11/1 -> Terminator13/1  "HIL_Iabc_Sec"
  [A7] -> Controlled Voltage Source3/1
  Demux3/1 -> [A7]
  [VabcgridSec] -> Data Type Conversion13/1
  Demux3/3 -> [A5]
  "Power (3ph, Instantaneous)"/1 -> Mux/1
  "Power (3ph, Instantaneous)"/2 -> Mux/2
  Three-Phase V-I Measurement4/2 -> [IabcgridSec]
  [A_TOP] -> Mosfet/1
  [C_TOP] -> Mosfet2/1
  [B_TOP] -> Mosfet1/1
  [B_BOT] -> Mosfet4/1
  [C_BOT] -> Mosfet5/1
  [A_BOT] -> Mosfet3/1
  Test/1 -> [Test]  "Test"
  PWM_Duty/1 -> Demux/1  "HIL_PWM"
  Demux/1 -> [A_TOP]
  Demux/2 -> [A_BOT]
  Demux/5 -> [C_TOP]
  Demux/4 -> [B_BOT]
  Demux/3 -> [B_TOP]
  Demux/6 -> [C_BOT]
  connections:
  Voltage Measurement1/LConn1 -- R_Passive1/LConn1 -- Mosfet/LConn1 -- Mosfet1/LConn1 -- Mosfet2/LConn1 -- R_Battery1/RConn1 -- C3/LConn1
  Ground2/LConn1 -- Mosfet3/RConn1 -- Mosfet4/RConn1 -- Mosfet5/RConn1 -- R_Passive1/RConn1 -- Battery1/LConn1 -- C4/RConn1 -- Voltage Measurement1/LConn2
  Three-Phase Transformer (Two Windings)1/RConn2 -- Three-Phase V-I Measurement4/LConn2
  Three-Phase V-I Measurement4/RConn3 -- Controlled Voltage Source5/RConn1
  C4/LConn1 -- C3/RConn1
  Three-Phase Transformer (Two Windings)1/LConn3 -- Three-Phase V-I Measurement2/RConn3
  Three-Phase Transformer (Two Windings)1/RConn1 -- Three-Phase V-I Measurement4/LConn1
  Three-Phase V-I Measurement2/RConn2 -- Three-Phase Transformer (Two Windings)1/LConn2
  L1 = 2 mH L1_esr = 1 Ohm1/RConn1 -- Three-Phase V-I Measurement2/LConn1
  Three-Phase V-I Measurement3/RConn1 -- L1 = 2 mH L1_esr = 1 Ohm1/LConn1
  Three-Phase V-I Measurement3/RConn2 -- L2 = 2 mH L2_esr = 1 Ohm1/LConn1
  L3 = 2 mH L3_esr = 1 Ohm1/RConn1 -- Three-Phase V-I Measurement2/LConn3
  Battery1/RConn1 -- R_Battery1/LConn1
  Three-Phase Transformer (Two Windings)1/LConn1 -- Three-Phase V-I Measurement2/RConn1
  Three-Phase V-I Measurement4/RConn2 -- Controlled Voltage Source4/RConn1
  Three-Phase V-I Measurement3/RConn3 -- L3 = 2 mH L3_esr = 1 Ohm1/LConn1
  Three-Phase Transformer (Two Windings)1/RConn3 -- Three-Phase V-I Measurement4/LConn3
  Three-Phase V-I Measurement4/RConn1 -- Controlled Voltage Source3/RConn1
  Three-Phase V-I Measurement2/LConn2 -- L2 = 2 mH L2_esr = 1 Ohm1/RConn1
  Controlled Voltage Source5/LConn1 -- Ground4/LConn1 -- Controlled Voltage Source4/LConn1 -- Controlled Voltage Source3/LConn1
  Mosfet2/RConn1 -- Three-Phase V-I Measurement3/LConn3 -- Mosfet5/LConn1
  Mosfet4/LConn1 -- Three-Phase V-I Measurement3/LConn2 -- Mosfet1/RConn1
  Mosfet/RConn1 -- Three-Phase V-I Measurement3/LConn1 -- Mosfet3/LConn1

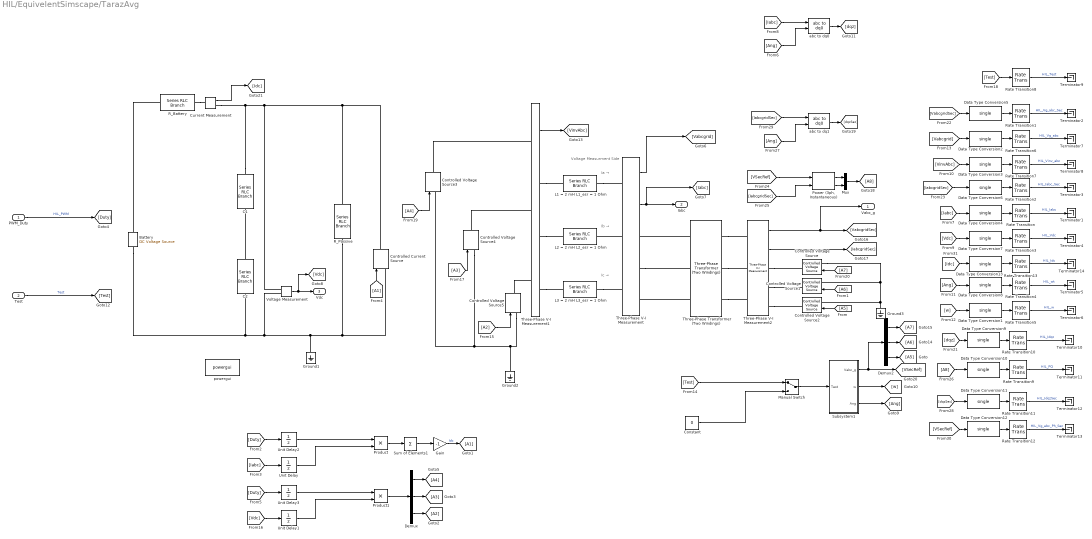
== system HIL/EquivelentSimscape/TarazAvg ==
  note: Voltage
      | Measurment
      | Side
  note: Ia
      | →
  note: Ib
      | →
  note: Ic
      | →
  PWM_Duty : Inport
  Test : Inport  Port=2
  Battery : spsDCVoltageSourceLib/DC Voltage Source  Amplitude=Hil.HVDC_V  Measurements=None
  C1 : spsSeriesRLCBranchLib/Series RLC Branch  LConnTagsString=__new0  RConnTagsString=__new0  BranchType=RLC  Resistance=Hil.HVDC_Cesr  Inductance=Hil.HVDC_Cesl  SetiL0=off  InitialCurrent=0  Capacitance=Hil.HVDC_C/2  Setx0=off  InitialVoltage=0  Measurements=None
  C2 : spsSeriesRLCBranchLib/Series RLC Branch  LConnTagsString=__new0  RConnTagsString=__new0  BranchType=RLC  Resistance=Hil.HVDC_Cesr  Inductance=Hil.HVDC_Cesl  SetiL0=off  InitialCurrent=0  Capacitance=Hil.HVDC_C/2  Setx0=off  InitialVoltage=0  Measurements=None
  Constant : Constant  Value=0  OutDataTypeStr=boolean
  Controlled Current Source : spsControlledCurrentSourceLib/Controlled Current Source  Initialize=on  Source_Type=AC  Amplitude=0  Phase=0  Frequency=0  Measurements=None
  Controlled Voltage Source{,1..5} (6 alike) : spsControlledVoltageSourceLib/Controlled Voltage Source  Initialize=on  Source_Type=AC  Amplitude=0  Phase=0  Frequency=0  Measurements=None
  Current Measurement : spsCurrentMeasurementLib/Current Measurement  PhasorSimulation=off  OutputType=Complex  PSBequivalent=0
  Data Type Conversion{1..13} (13 alike) : DataTypeConversion  OutDataTypeStr=single  SaturateOnIntegerOverflow=off  RndMeth=Floor
  Demux : Demux  Outputs=3
  Demux2 : Demux  Outputs=3
  Gain : Gain  Gain=-1
  Ground1 : spsGroundLib/Ground  LConnTagsString=a
  Ground2 : spsGroundLib/Ground  LConnTagsString=a
  Ground3 : spsGroundLib/Ground  LConnTagsString=a
  L1 = 2 mH L1_esr = 1 Ohm : spsSeriesRLCBranchLib/Series RLC Branch  LConnTagsString=__new0  RConnTagsString=__new0  BranchType=RL  Resistance=Hil.Inductor_R  Inductance=Hil.Inductor_L  SetiL0=off  InitialCurrent=0  Capacitance=1e-6  Setx0=off  InitialVoltage=0  Measurements=None
  L2 = 2 mH L2_esr = 1 Ohm : spsSeriesRLCBranchLib/Series RLC Branch  LConnTagsString=__new0  RConnTagsString=__new0  BranchType=RL  Resistance=Hil.Inductor_R  Inductance=Hil.Inductor_L  SetiL0=off  InitialCurrent=0  Capacitance=1e-6  Setx0=off  InitialVoltage=0  Measurements=None
  L3 = 2 mH L3_esr = 1 Ohm : spsSeriesRLCBranchLib/Series RLC Branch  LConnTagsString=__new0  RConnTagsString=__new0  BranchType=RL  Resistance=Hil.Inductor_R  Inductance=Hil.Inductor_L  SetiL0=off  InitialCurrent=0  Capacitance=1e-6  Setx0=off  InitialVoltage=0  Measurements=None
  Manual Switch : ManualSwitch
  Mux : Mux  Inputs=2
  "Power (3ph, Instantaneous)" : spsPower3phInstantaneousLib/Power (3ph, Instantaneous)
  Product : Product
  Product1 : Product
  R_Battery : spsSeriesRLCBranchLib/Series RLC Branch  LConnTagsString=__new0  RConnTagsString=__new0  BranchType=R  Resistance=Hil.HVDC_Vesr  Inductance=Hil.HVDC_Vesl  SetiL0=off  InitialCurrent=0  Capacitance=1e-6  Setx0=off  InitialVoltage=0  Measurements=None
  R_Passive : spsSeriesRLCBranchLib/Series RLC Branch  LConnTagsString=__new0  RConnTagsString=__new0  BranchType=R  Resistance=Hil.HVDC_Rpasiv  Inductance=1e-3  SetiL0=off  InitialCurrent=0  Capacitance=1e-6  Setx0=off  InitialVoltage=0  Measurements=None
  Rate Transition{,1..2,4,6..7,12} (7 alike) : RateTransition  OutPortSampleTime=Hil.MeasFastSmplTime
  Rate Transition{3,5,8..11,13} (7 alike) : RateTransition  OutPortSampleTime=Hil.MeasSlowSmplTime
  Subsystem1 : Subsystem
  Sum of Elements1 : Sum  Inputs=+
  Terminator{1..14} (14 alike) : Terminator
  Three-Phase Transformer (Two Windings) : spsThreePhaseTransformerTwoWindingsLib/Three-Phase Transformer (Two Windings)  Winding1Connection=Y  Winding2Connection=Delta (D1)  CoreType=Three single-phase transformers  SetSaturation=off  Hysteresis=off  DataFile='hysteresis'  SetInitialFlux=off  Measurements=None  UNITS=SI  NominalPower=[ 100e3 , 50 ]  Winding1=[100 Hil.Transformer_R1 Hil.Transformer_L1]  Winding2=[(Hil.Transformer_N )*100 Hil.Transformer_R2 Hil.Transformer_L2]  Rm=Hil.Transformer_Rc  Lm=Hil.Transformer_Lm  L0=0.5  Saturation=[0 0;1.1327 0.53955;471.96 0.68343]  InitialFluxes=[0.3597 -0.3597 0.31474]  BreakLoop=off  DiscreteSolver=Trapezoidal iterative  DataType=on  TransfoNumber=1
  Three-Phase V-I Measurement : spsThreePhaseVIMeasurementLib/Three-Phase V-I Measurement  VoltageMeasurement=phase-to-phase  SetLabelV=off  LabelV=Vabc  Vpu=off  VpuLL=off  CurrentMeasurement=yes  SetLabelI=off  LabelI=Iabc  Ipu=off  Pbase=100e6  Vbase=500e3  OutputType=Complex  PhasorSimulation=off  PSBequivalent=0
  Three-Phase V-I Measurement1 : spsThreePhaseVIMeasurementLib/Three-Phase V-I Measurement  VoltageMeasurement=phase-to-ground  SetLabelV=off  LabelV=Vabc  Vpu=off  VpuLL=off  CurrentMeasurement=no  SetLabelI=off  LabelI=Iabc  Ipu=off  Pbase=100e6  Vbase=500e3  OutputType=Complex  PhasorSimulation=off  PSBequivalent=0
  Three-Phase V-I Measurement2 : spsThreePhaseVIMeasurementLib/Three-Phase V-I Measurement  VoltageMeasurement=phase-to-phase  SetLabelV=off  LabelV=Vabc  Vpu=off  VpuLL=off  CurrentMeasurement=yes  SetLabelI=off  LabelI=Iabc  Ipu=off  Pbase=100e6  Vbase=500e3  OutputType=Complex  PhasorSimulation=off  PSBequivalent=0
  Unit Delay{,1..3} (4 alike) : UnitDelay  SampleTime=-1  HasFrameUpgradeWarning=on
  Voltage Measurement : spsVoltageMeasurementLib/Voltage Measurement  PhasorSimulation=off  OutputType=Complex  PSBequivalent=0
  abc to dq0 : spsabctodq0Lib/abc to dq0  Alignment=Aligned with phase A axis
  abc to dq1 : spsabctodq0Lib/abc to dq0  Alignment=Aligned with phase A axis
  powergui : spspowerguiLib/powergui  Priority=1  SimulationMode=Discrete  SampleTime=Sim.ContSampleTime  frequency=60  Iterations=50  frequencyindice=0  Pbase=100e6  ErrMax=1e-4  UnitsV=kV  UnitsW=MW  buscounter=0  FunctionMessages=off  echomessages=off  EnableUseOfTLC=off  CurrentSourceSwitches=off  DisableSnubberDevices=off  DisableRonSwitches=off  DisableVfSwitches=off  DisplayEquations=off  AutomaticDiscreteSolvers=off  SolverType=Tustin/Backward Euler (TBE)  Interpol=off  ExternalGateDelay=off  methode=off  Ts=100  x0status=blocks  SPID=on  SwTol=0  HookPort=off  NonlinearTolerance=1e-4  nMaxIteration=100  ContinueOnMaxIteration=off  RestoreLinks=warning  ResistiveCurrentMeasurement=off  Frange=[0:2:500]  Ylog=off  Xlog=on  ShowGrid=off  save=off  variable=ZData  structure=0  ZoomFFT=off  StartTime=0.0  cycles=1  DisplayStyle=1  fundamental=60  FreqAxis=off  MaxFrequency=1000  frequencyindicesteady=1  RmsSteady=1  display=off
  Vabc_g : Outport
  Iabc : Outport  Port=2
  Vdc : Outport  Port=3
  wires:
  [Idc] -> Data Type Conversion13/1
  Rate Transition13/1 -> Terminator14/1  "HIL_Idc"
  Data Type Conversion13/1 -> Rate Transition13/1
  Current Measurement/1 -> [Idc]
  [VSecRef] -> Data Type Conversion12/1
  Data Type Conversion12/1 -> Rate Transition12/1
  Rate Transition12/1 -> Terminator13/1  "HIL_Vg_abc_Ph_Sec"
  [dqzSec] -> Data Type Conversion11/1
  Rate Transition11/1 -> Terminator12/1  "HIL_IdqzSec"
  Data Type Conversion11/1 -> Rate Transition11/1
  [IabcgridSec] -> abc to dq1/1
  abc to dq1/1 -> [dqzSec]
  [Ang] -> abc to dq1/2
  [A8] -> Data Type Conversion10/1
  Mux/1 -> [A8]
  Rate Transition9/1 -> Terminator11/1  "HIL_PQ"
  Data Type Conversion10/1 -> Rate Transition9/1
  "Power (3ph, Instantaneous)"/2 -> Mux/2
  "Power (3ph, Instantaneous)"/1 -> Mux/1
  [IabcgridSec] -> "Power (3ph, Instantaneous)"/2
  [VSecRef] -> "Power (3ph, Instantaneous)"/1
  [IabcgridSec] -> Data Type Conversion6/1
  Rate Transition2/1 -> Terminator3/1  "HIL_Iabc_Sec"
  Data Type Conversion6/1 -> Rate Transition2/1
  [VabcgridSec] -> Data Type Conversion5/1
  Rate Transition1/1 -> Terminator2/1  "HIL_Vg_abc_Sec"
  Data Type Conversion5/1 -> Rate Transition1/1
  Three-Phase V-I Measurement2/2 -> [IabcgridSec]
  Three-Phase V-I Measurement2/1 -> [VabcgridSec], Vabc_g/1
  [A7] -> Controlled Voltage Source/1
  Demux2/1 -> [A7]
  [A6] -> Controlled Voltage Source1/1
  Demux2/2 -> [A6]
  [A5] -> Controlled Voltage Source2/1
  Demux2/3 -> [A5]
  [Test] -> Manual Switch/1
  Constant/1 -> Manual Switch/2
  Unit Delay3/1 -> Product1/1
  Unit Delay2/1 -> Product/1
  Subsystem1/3(Ang) -> [Ang]
  Subsystem1/2(w) -> [w]
  Manual Switch/1 -> Subsystem1/1(Test)
  Three-Phase V-I Measurement1/1 -> [VinvAbc]
  Test/1 -> [Test]  "Test"
  Three-Phase V-I Measurement/1 -> [Vabcgrid]
  Three-Phase V-I Measurement/2 -> [Iabc], Iabc/1
  Voltage Measurement/1 -> [Vdc], Vdc/1
  PWM_Duty/1 -> [Duty]  "HIL_PWM"
  [Vdc] -> Data Type Conversion7/1
  [dqz] -> Data Type Conversion9/1
  Data Type Conversion9/1 -> Rate Transition10/1
  Rate Transition8/1 -> Terminator9/1  "HIL_Test"
  Data Type Conversion2/1 -> Rate Transition6/1
  [Test] -> Rate Transition8/1
  [VinvAbc] -> Data Type Conversion3/1
  Data Type Conversion4/1 -> Rate Transition/1
  Data Type Conversion8/1 -> Rate Transition4/1
  Data Type Conversion3/1 -> Rate Transition7/1
  Rate Transition6/1 -> Terminator7/1  "HIL_Vg_abc"
  [Vabcgrid] -> Data Type Conversion2/1
  Rate Transition7/1 -> Terminator8/1  "HIL_Vinv_abc"
  Data Type Conversion1/1 -> Rate Transition5/1
  [Ang] -> Data Type Conversion8/1
  Rate Transition4/1 -> Terminator5/1  "HIL_wt"
  Rate Transition10/1 -> Terminator10/1  "HIL_Idqz"
  Data Type Conversion7/1 -> Rate Transition3/1
  Rate Transition3/1 -> Terminator4/1  "HIL_Vdc"
  [Iabc] -> Data Type Conversion4/1
  Rate Transition/1 -> Terminator1/1  "HIL_Iabc"
  [w] -> Data Type Conversion1/1
  Rate Transition5/1 -> Terminator6/1  "HIL_w"
  [Ang] -> abc to dq0/2
  abc to dq0/1 -> [dqz]
  [Iabc] -> abc to dq0/1
  Subsystem1/1(Vabc_g) -> Demux2/1, [VSecRef]
  [Duty] -> Unit Delay2/1
  [Iabc] -> Unit Delay/1
  Product/1 -> Sum of Elements1/1
  Unit Delay/1 -> Product/2
  Sum of Elements1/1 -> Gain/1
  Gain/1 -> [A1]  "Idc"
  [A1] -> Controlled Current Source/1
  Unit Delay1/1 -> Product1/2
  Product1/1 -> Demux/1
  [Vdc] -> Unit Delay1/1
  [Duty] -> Unit Delay3/1
  Demux/3 -> [A2]
  [A2] -> Controlled Voltage Source5/1
  Demux/2 -> [A3]
  [A3] -> Controlled Voltage Source4/1
  Demux/1 -> [A4]
  [A4] -> Controlled Voltage Source3/1
  connections:
  R_Battery/RConn1 -- Current Measurement/LConn1
  C1/LConn1 -- Current Measurement/RConn1 -- Voltage Measurement/LConn1 -- Controlled Current Source/RConn1 -- R_Passive/LConn1
  Three-Phase V-I Measurement2/RConn1 -- Controlled Voltage Source/RConn1
  Three-Phase V-I Measurement2/RConn2 -- Controlled Voltage Source1/RConn1
  Three-Phase V-I Measurement2/RConn3 -- Controlled Voltage Source2/RConn1
  Three-Phase Transformer (Two Windings)/RConn3 -- Three-Phase V-I Measurement2/LConn3
  Three-Phase Transformer (Two Windings)/RConn2 -- Three-Phase V-I Measurement2/LConn2
  Three-Phase Transformer (Two Windings)/RConn1 -- Three-Phase V-I Measurement2/LConn1
  Battery/RConn1 -- R_Battery/LConn1
  Three-Phase V-I Measurement1/RConn3 -- L3 = 2 mH L3_esr = 1 Ohm/LConn1
  Three-Phase V-I Measurement1/RConn2 -- L2 = 2 mH L2_esr = 1 Ohm/LConn1
  Three-Phase V-I Measurement1/RConn1 -- L1 = 2 mH L1_esr = 1 Ohm/LConn1
  C2/LConn1 -- C1/RConn1
  R_Passive/RConn1 -- Voltage Measurement/LConn2 -- Battery/LConn1 -- C2/RConn1 -- Ground1/LConn1 -- Controlled Current Source/LConn1
  Three-Phase V-I Measurement/LConn2 -- L2 = 2 mH L2_esr = 1 Ohm/RConn1
  L3 = 2 mH L3_esr = 1 Ohm/RConn1 -- Three-Phase V-I Measurement/LConn3
  L1 = 2 mH L1_esr = 1 Ohm/RConn1 -- Three-Phase V-I Measurement/LConn1
  Three-Phase Transformer (Two Windings)/LConn3 -- Three-Phase V-I Measurement/RConn3
  Three-Phase V-I Measurement/RConn2 -- Three-Phase Transformer (Two Windings)/LConn2
  Three-Phase Transformer (Two Windings)/LConn1 -- Three-Phase V-I Measurement/RConn1
  Controlled Voltage Source2/LConn1 -- Ground3/LConn1 -- Controlled Voltage Source1/LConn1 -- Controlled Voltage Source/LConn1
  Controlled Voltage Source5/RConn1 -- Three-Phase V-I Measurement1/LConn3
  Controlled Voltage Source4/RConn1 -- Three-Phase V-I Measurement1/LConn2
  Three-Phase V-I Measurement1/LConn1 -- Controlled Voltage Source3/RConn1
  Controlled Voltage Source4/LConn1 -- Controlled Voltage Source5/LConn1 -- Ground2/LConn1 -- Controlled Voltage Source3/LConn1
